simulink model "pathNavigation_Logic_start"  (R2017a)
settings: Solver=FixedStepDiscrete  StartTime=0.0  StopTime=inf  FixedStep=0.01  RelTol=1e-3
PreLoadFcn:
  | robotParameters;
  | load examplePathNavigationMap;
undefined symbols (not defined in the file or in its folder): axleLength, motorIp, motorSp, ticksPerRot, wheelR
libraries: mobileRoboticsTrainingLib x7, simulink_extras x1
settings Model: Creator=sseshadr  LastModifiedBy=shiremat

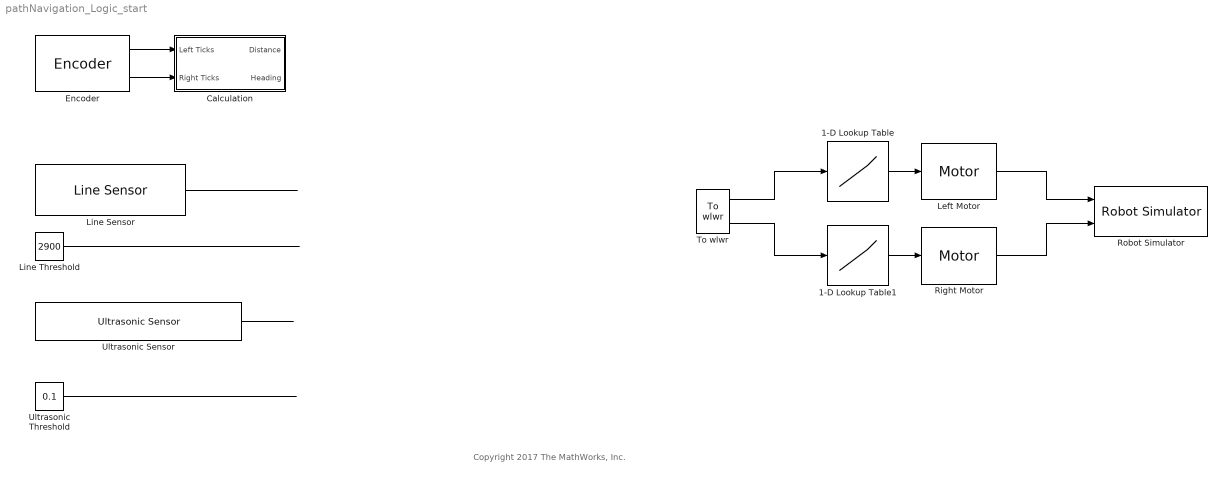
== system pathNavigation_Logic_start ==
  note: Copyright 2017 The MathWorks, Inc.
  1-D Lookup Table : Lookup_n-D  NumberOfTableDimensions=1  BreakpointsForDimension1=motorSp  Table=motorIp  ExtrapMethod=Clip  InternalRulePriority=Speed  RndMeth=Simplest  InputSameDT=on
  1-D Lookup Table1 : Lookup_n-D  NumberOfTableDimensions=1  BreakpointsForDimension1=motorSp  Table=motorIp  ExtrapMethod=Clip  InternalRulePriority=Speed  RndMeth=Simplest  InputSameDT=on
  Calculation : Subsystem
  Encoder : mobileRoboticsTrainingLib/Encoder  axleLength=axleLength  wheelR=wheelR  ticksPerRot=ticksPerRot
      settings: SourceProductName=Mobile Robotics Training Library
  Left Motor : mobileRoboticsTrainingLib/Motor  motorPlant=wheelMotorModel  sensorType=Speed
      settings: SourceProductName=Mobile Robotics Training Library
  Line Sensor : mobileRoboticsTrainingLib/Line Sensor  mapVariable=mapForSim  envVal=2850  lineVal=2950  sensOff=[0.01 0]
      settings: SourceProductName=Mobile Robotics Training Library
  Line Threshold : Constant  Value=2900
  Right Motor : mobileRoboticsTrainingLib/Motor  motorPlant=wheelMotorModel  sensorType=Speed
      settings: SourceProductName=Mobile Robotics Training Library
  Robot Simulator : mobileRoboticsTrainingLib/Robot Simulator  Priority=99  mapVar=mapForSim  startX=0.5  startY=0.25  startTheta=90  axleLength=axleLength  wheelR=wheelR
  To wlwr : mobileRoboticsTrainingLib/To wlwr  axleLength=axleLength  wheelR=wheelR
  Ultrasonic Sensor : mobileRoboticsTrainingLib/Ultrasonic Sensor  mapVar=mapForSim  maxSenRange=0.25  minSenRange=0.02  senRes=0.01  sensOff=[0 0]
      settings: SourceProductName=Mobile Robotics Training Library
  Ultrasonic Threshold : Constant  Value=0.1
  wires:
  Left Motor/1 -> Robot Simulator/1
  1-D Lookup Table1/1 -> Right Motor/1
  1-D Lookup Table/1 -> Left Motor/1
  Right Motor/1 -> Robot Simulator/2
  To wlwr/1 -> 1-D Lookup Table/1
  To wlwr/2 -> 1-D Lookup Table1/1
  ? -> To wlwr/1
  ? -> To wlwr/2
  Ultrasonic Sensor/1 -> ?
  Line Sensor/1 -> ?
  Line Threshold/1 -> ?
  Ultrasonic Threshold/1 -> ?
  Encoder/1 -> Calculation/1(Left Ticks)
  Encoder/2 -> Calculation/2(Right Ticks)

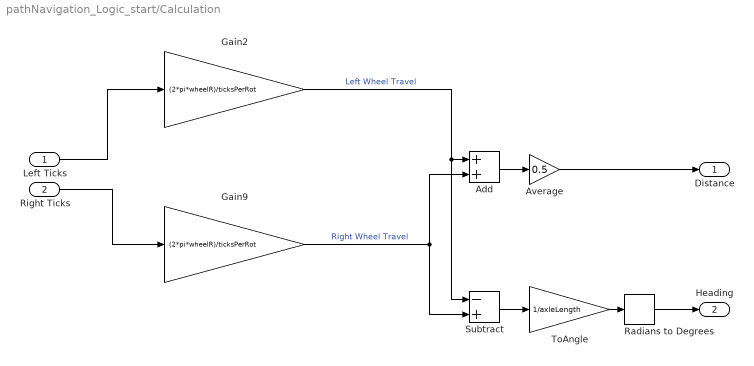
== system pathNavigation_Logic_start/Calculation ==
  Left Ticks : Inport
  Right Ticks : Inport  Port=2
  Add : Sum
  Average : Gain  Gain=0.5
  Gain2 : Gain  Gain=(2*pi*wheelR)/ticksPerRot
  Gain9 : Gain  Gain=(2*pi*wheelR)/ticksPerRot
  Radians to Degrees : simulink_extras/Transformations/Radians to Degrees
  Subtract : Sum  Inputs=-+
  ToAngle : Gain  Gain=1/axleLength
  Distance : Outport
  Heading : Outport  Port=2
  wires:
  Average/1 -> Distance/1
  Add/1 -> Average/1
  Gain2/1 -> Subtract/1, Add/1  "Left Wheel Travel"
  Right Ticks/1 -> Gain9/1
  Left Ticks/1 -> Gain2/1
  Gain9/1 -> Subtract/2, Add/2  "Right Wheel Travel"
  Subtract/1 -> ToAngle/1
  ToAngle/1 -> Radians to Degrees/1
  Radians to Degrees/1 -> Heading/1
